simulink model "LKAS_AutoSave_DF_20211230_1703"  (R2018b)
settings: Solver=FixedStepDiscrete  StartTime=0.0  StopTime=10.0  FixedStep=0.01  RelTol=1e-3
InitFcn:
  | tmpVer = ver('MATLAB');
  | tmpVer = str2num(tmpVer.Version);
  | % -------------------------------------------------------------------
  | %  MATLAB file generated by Simulink.saveVars on 21-Nov-2019 10:06:14
  | %  MATLAB version: 7.13.0.564 (R2011b)
  | % -------------------------------------------------------------------
  | 
  | 
  | SInt16 = Simulink.AliasType;
  | SInt16.Description = 'Num';
  | if (tmpVer > 7.11)
  | 	SInt16.DataScope = 'Auto';
  | end
  | SInt16.HeaderFile = 'Rte_Type.h';
  | SInt16.BaseType = 'int16';
  | 
  | SInt32 = Simulink.AliasType;
  | SInt32.Description = 'Num';
  | if (tmpVer > 7.11)
  | 	SInt32.DataScope = 'Auto';
  | end
  | SInt32.HeaderFile = 'Rte_Type.h';
  | SInt32.BaseType = 'int32';
  | 
  | SInt8 = Simulink.AliasType;
  | SInt8.Description = 'Num';
  | if (tmpVer > 7.11)
  | 	SInt8.DataScope = 'Auto';
  | end
  | SInt8.HeaderFile = 'Rte_Type.h';
  | SInt8.BaseType = 'int8';
  | 
  | T_A_m2_1024_1_u32 = Simulink.NumericType;
  | T_A_m2_1024_1_u32.Description = 'm2 (square meters  (m2))';
  | if (tmpVer > 7.11)
  | 	T_A_m2_1024_1_u32.DataScope = 'Auto';
  | end
  | T_A_m2_1024_1_u32.HeaderFile = 'Rte_Type.h';
  | T_A_m2_1024_1_u32.DataTypeMode = 'Fixed-point: slope and bias scaling';
  | T_A_m2_1024_1_u32.SignednessBool = false;
  | T_A_m2_1024_1_u32.WordLength = 32;
  | T_A_m2_1024_1_u32.FixedExponent = -10;
  | T_A_m2_1024_1_u32.SlopeAdjustmentFactor = 1;
  | T_A_m2_1024_1_u32.Bias = 0;
  | T_A_m2_1024_1_u32.DataTypeOverride = 'Inherit';
  | T_A_m2_1024_1_u32.IsAlias = true;
  | 
  | T_A_m2_65536_1_u16 = Simulink.NumericType;
  | T_A_m2_65536_1_u16.Description = 'm2 (square meters  (m2))';
  | if (tmpVer > 7.11)
  | 	T_A_m2_65536_1_u16.DataScope = 'Auto';
  | end
  | T_A_m2_65536_1_u16.HeaderFile = 'Rte_Type.h';
  | T_A_m2_65536_1_u16.DataTypeMode = 'Fixed-point: slope and bias scaling';
  | T_A_m2_65536_1_u16.SignednessBool = false;
  | T_A_m2_65536_1_u16.WordLength = 16;
  | T_A_m2_65536_1_u16.FixedExponent = -16;
  | T_A_m2_65536_1_u16.SlopeAdjustmentFactor = 1;
  | T_A_m2_65536_1_u16.Bias = 0;
  | T_A_m2_65536_1_u16.DataTypeOverride = 'Inherit';
  | ... (+4647 lines)
StopFcn:
  | clear  T_A_m2_1024_1_u32 T_A_m2_65536_1_u16 T_A_m2_Float32 T_A_mm2_10_1_u16 T_A_mm2_4_1_s16 T_A_mm2_Float32 T_Cnt_Num_10_1_u32 T_Cnt_Num_1_1_s16 T_Cnt_Num_1_1_s32 T_Cnt_Num_1_1_s8 T_Cnt_Num_1_1_u16 T_Cnt_Num_1_1_u32 T_Cnt_Num_1_1_u8 T_E_J_1_1_s32 T_E_J_Float32 T_E_kJ_128_1_s32 T_E_kJ_Float32 T_E_kwh_10_1_u16 T_E_kwh_Float32 T_Epl_kwhpkm_100_1_u16 T_Epl_kwhpkm_Float32 T_F_N_1_1_s16 T_F_N_Float32 T_I_A_1000_1_u16 T_I_A_1048576_1_s32 T_I_A_2048_1_s16 T_I_A_32_1_s16 T_I_A_Float32 T_I_mA_1_1_s16 T_I_mA_32768_128_s16 T_I_mA_Float32 T_J_kgpm2_128_1_u16 T_J_kgpm2_Float32 T_K_NA_1000_1_s16 T_K_NA_100_1_s16 T_K_NA_100_1_u16 T_K_NA_1024_1_s16 T_K_NA_1024_1_u16 T_K_NA_128_1_s16 T_K_NA_128_1_u16 T_K_NA_128_1_u8 T_K_NA_16777216_1_u32 T_K_NA_16_1_s16 T_K_NA_16_1_u16 T_K_NA_16_1_u8 T_K_NA_1_16_u16 T_K_NA_1_1_s16 T_K_NA_1_1_u16 T_K_NA_1_1_u8 T_K_NA_32768_1_s16 T_K_NA_32768_1_u16 T_K_NA_32_1_s8 T_K_NA_4096_1_u16 T_K_NA_4194304_1_s32 T_K_NA_4194304_1_u16 T_K_NA_65536_1_s32 T_K_NA_65536_1_u16 T_K_NA_8192_1_s16 T_K_NA_8_1_s16 T_K_NA_Float32 T_M_Nm_16_1_s16 T_M_Nm_1_1_s16 T_M_Nm_32768_1_s16 T_M_Nm_32_1_s16 T_M_Nm_4_1_s16 T_M_Nm_512_1_s16 T_M_Nm_Float32 T_P_W_1_4_s16 T_P_W_1_8_s16 T_P_W_Float32 T_P_kW_128_1_s16 T_P_kW_1_8_s16 T_P_kW_8_1_s32 T_P_kW_Float32 T_Pct_pct_1024_1_s32 T_Pct_pct_1024_1_u32 T_Pct_pct_10_1_s16 T_Pct_pct_10_1_u32 T_Pct_pct_128_100_s8 T_Pct_pct_1_1_s16 T_Pct_pct_1_4_u8 T_Pct_pct_255_100_u16 T_Pct_pct_255_100_u8 T_Pct_pct_256_1_s16 T_Pct_pct_256_1_u16 T_Pct_pct_65535_100_u16 T_Pct_pct_Float32 T_R_ohm_1024_1_s16 T_R_ohm_32_1_s16 T_R_ohm_Float32 T_TK_K_16_1_s16 T_TK_K_Float32 T_T_degC_10_400_1_u16 T_T_degC_16_1_s16 T_T_degC_1_40_1_u8 T_T_degC_2_80_1_u8 T_T_degC_Float32 T_U_V_1000_1_u16 T_U_V_10_1_u8 T_U_V_200_1_u8 T_U_V_32_1_s16 T_U_V_4096_1_s16 T_U_V_512_1_s16 T_U_V_65535_8_u16 T_U_V_8192_1_u16 T_U_V_Float32 T_U_mV_1_1_s16 T_U_mV_256_20_u16 T_U_mV_Float32 T_V_l_256_1_s16 T_V_l_4096_1_s16 T_V_l_64_1_s16 T_V_l_65535_100_u16 T_V_l_Float32 T_V_ml_128_1_s16 T_V_ml_1_1_s16 T_V_ml_32768_1_s16 T_V_ml_Float32 T_V_ul_32_1_u16 T_V_ul_Float32 T_Vpl_clpkm_512_1_u16 T_Vpl_clpkm_Float32 T_a_kphps_16_1_s16 T_a_kphps_Float32 T_a_mps2_128_1_s16 T_a_mps2_Float32 T_c_MJpkg_256_1_s16 T_c_MJpkg_Float32 T_c_kJpgpK_1024_1_s16 T_c_kJpgpK_Float32 T_c_kJpkgpK_128_1_u16 T_c_kJpkgpK_Float32 T_chrg_Ah_1_1_s16 T_chrg_Ah_1_1_u16 T_chrg_Ah_1_1_u8 T_chrg_Ah_256_1_u16 T_chrg_Ah_4194304_1_s32 T_chrg_Ah_512_1_u16 T_chrg_Ah_8_1_u16 T_chrg_Ah_Float32 T_cmp_NA_100_1_s16 T_cmp_NA_128_1_s16 T_cmp_NA_16_1_s16 T_cmp_NA_32768_1_u16 T_cmp_NA_Float32 T_d2n_rpmps2_4_1_s16 T_d2n_rpmps2_Float32 T_dPct_pctps_16_1_s16 T_dPct_pctps_256_1_s16 T_dPct_pctps_Float32 T_dT_degCps_128_1_s16 T_dT_degCps_Float32 T_dV_lph_1_1_s16 T_dV_lph_Float32 T_dV_lpm_128_1_s16 T_dV_lpm_32_1_s16 T_dV_lpm_Float32 T_dV_lps_1024_1_u16 T_dV_lps_4_1_u16 T_dV_lps_Float32 T_dV_mlps_1024_1_s16 T_dV_mlps_Float32 T_d_BitField16 T_dm_gps_128_1_s16 T_dm_gps_128_1_u16 T_dm_gps_256_1_u16 T_dm_gps_Float32 T_dm_mgps_1_1_s16 T_dm_mgps_Float32 T_dn_rpmps_1_1_s16 T_dn_rpmps_2_1_s16 T_dn_rpmps_Float32 T_dp_Paps_1_1_s16 T_dp_Paps_Float32 T_dp_kPaps_1_1_s16 T_dp_kPaps_8_1_s16 T_dp_kPaps_Float32 T_dphi_degps_128_1_s16 T_dphi_degps_8_1_s16 T_dphi_degps_Float32 T_dr_ps_256_1_s16 T_dr_ps_Float32 T_drho_mgplps_1_2_s16 T_drho_mgplps_Float32 T_e_NA_1_1_u8 T_f_Hz_1_1_u16 T_f_Hz_1_1_u32 T_f_Hz_64_1_u16 T_f_Hz_8_1_s16 T_f_Hz_Float32 T_g_BitField32 T_l_km_16_1_s16 T_l_km_1_1_u16 T_l_km_1_1_u32 T_l_km_Float32 T_l_m_1024_1_s16 T_l_m_16_1_s16 T_l_m_1_1_u32 T_l_m_Float32 T_l_mm_16_1_s16 T_l_mm_1_1_u16 T_l_mm_4096_1_s16 T_l_mm_4_1_u8 T_l_mm_64_1_s16 T_l_mm_Float32 T_m_g_1_1_s16 T_m_g_2048_1_s16 T_m_g_32_1_u16 T_m_g_Float32 T_m_kg_1024_1_s16 T_m_kg_1_1_s16 T_m_kg_1_1_u32 T_m_kg_Float32 T_m_mg_128_1_s16 T_m_mg_32_1_s16 T_m_mg_Float32 T_n_rpm_1_1_s16 T_n_rpm_1_25_u8 T_n_rpm_256_50_u16 T_n_rpm_2_25_u8 T_n_rpm_4_1_u16 T_n_rpm_Float32 T_p_MPa_64_1_s16 T_p_MPa_Float32 T_p_Pa_1_1_s16 T_p_Pa_Float32 T_p_kPa_1_10_u16 T_p_kPa_1_1_s16 T_p_kPa_1_1_u8 T_p_kPa_256_1_u16 T_p_kPa_32_1_u16 T_p_kPa_64_1_s16 T_p_kPa_Float32 T_phi_deg_100_1_s16 T_phi_deg_1024_1_s16 T_phi_deg_128_1_s16 T_phi_deg_1_1_u8 T_phi_deg_256_1_s16 T_phi_deg_2_1_s8 T_phi_deg_32_1_s16 T_phi_deg_512_6_s32 T_phi_deg_Float32 T_phi_rad_2048_1_s16 T_phi_rad_Float32 T_r_NA_1024_1_s16 T_r_NA_1024_1_u16 T_r_NA_16384_1_s16 T_r_NA_16_1_s16 T_r_NA_256_1_s8 T_r_NA_256_1_u16 T_r_NA_32768_1_u16 T_r_NA_32_1_u16 T_r_NA_4096_1_s16 T_r_NA_65535_2_u16 T_r_NA_8192_1_u16 T_r_NA_Float32 T_rho_gpl_8192_1_s16 T_rho_gpl_Float32 T_rho_kgpm3_16_1_s16 T_rho_kgpm3_Float32 T_rho_mgpl_1_1_s16 T_rho_mgpl_64_1_s16 T_rho_mgpl_Float32 T_t_hour_1_1_s16 T_t_hour_Float32 T_t_m_1_1_u16 T_t_m_Float32 T_t_ms_1_1_s16 T_t_ms_1_1_u16 T_t_ms_1_1_u32 T_t_ms_4096_1_s16 T_t_ms_64_1_s16 T_t_ms_Float32 T_t_s_1000_1_s16 T_t_s_100_1_s16 T_t_s_10_1_s16 T_t_s_10_1_u16 T_t_s_1_1_s16 T_t_s_1_1_u16 T_t_s_1_1_u32 T_t_s_Float32 T_t_us_10_1_u32 T_t_us_1_1_s16 T_t_us_1_1_u32 T_t_us_1_4_u16 T_t_us_Float32 T_v_kph_1_1_u8 T_v_kph_64_1_s16 T_v_kph_64_1_u16 T_v_kph_Float32 T_v_mps_256_1_s16 T_v_mps_Float32 T_w_radps_32_1_s16 T_w_radps_Float32 T_y_BitField8 T_y_BitFieldDiagProgress T_y_BitFieldDiagStatus T_y_NA_1_1_u8 SInt16 SInt32 SInt8 T_BOOLEAN UInt16 UInt32 UInt8 s16 s32 s8 u16 u32 u8
model workspace (MAT data in the model file):
  MCOS : class17 (value not decoded)
  MCOS : class17 (value not decoded)
  MCOS : class17 (value not decoded)
  MCOS : class17 (value not decoded)
  MCOS : class17 (value not decoded)
  MCOS : class17 (value not decoded)
  MCOS : class17 (value not decoded)
  MCOS : class17 (value not decoded)
  MCOS : class17 (value not decoded)
  MCOS : class17 (value not decoded)
  MCOS : class17 (value not decoded)
  MCOS : class17 (value not decoded)
  MCOS : class17 (value not decoded)
  MCOS : class17 (value not decoded)
  MCOS : class17 (value not decoded)
  MCOS : class17 (value not decoded)
  MCOS : class17 (value not decoded)
  MCOS : class17 (value not decoded)
  MCOS : class17 (value not decoded)
  MCOS : class17 (value not decoded)
  MCOS : class17 (value not decoded)
  MCOS : class17 (value not decoded)
  MCOS : class17 (value not decoded)
  MCOS : class17 (value not decoded)
  MCOS : class17 (value not decoded)
  MCOS : class17 (value not decoded)
  MCOS : class17 (value not decoded)
  MCOS : class17 (value not decoded)
  MCOS : class17 (value not decoded)
  MCOS : class17 (value not decoded)
  MCOS : class17 (value not decoded)
  MCOS : class17 (value not decoded)
  MCOS : class17 (value not decoded)
  MCOS : class17 (value not decoded)
  MCOS : class17 (value not decoded)
  MCOS : class17 (value not decoded)
  MCOS : class17 (value not decoded)
  MCOS : class17 (value not decoded)
  MCOS : class17 (value not decoded)
  MCOS : class17 (value not decoded)
  MCOS : class17 (value not decoded)
  MCOS : class17 (value not decoded)
  MCOS : class17 (value not decoded)
  MCOS : class17 (value not decoded)
  MCOS : class17 (value not decoded)
  MCOS : class17 (value not decoded)
  MCOS : class17 (value not decoded)
  MCOS : class17 (value not decoded)
  MCOS : class17 (value not decoded)
  MCOS : class17 (value not decoded)
  MCOS : class17 (value not decoded)
  MCOS : class17 (value not decoded)
  MCOS : class17 (value not decoded)
  MCOS : class17 (value not decoded)
  MCOS : class17 (value not decoded)
  MCOS : class17 (value not decoded)
  MCOS : class17 (value not decoded)
  MCOS : class17 (value not decoded)
  MCOS : class17 (value not decoded)
  MCOS : class17 (value not decoded)
  MCOS : class17 (value not decoded)
  MCOS : class17 (value not decoded)
  MCOS : class17 (value not decoded)
  MCOS : class17 (value not decoded)
  MCOS : class17 (value not decoded)
  MCOS : class17 (value not decoded)
  MCOS : class17 (value not decoded)
  MCOS : class17 (value not decoded)
  MCOS : class17 (value not decoded)
  MCOS : class17 (value not decoded)
  MCOS : class17 (value not decoded)
  MCOS : class17 (value not decoded)
  MCOS : class17 (value not decoded)
  MCOS : class17 (value not decoded)
  MCOS : class17 (value not decoded)
  MCOS : class17 (value not decoded)
  MCOS : class17 (value not decoded)
  MCOS : class17 (value not decoded)
  MCOS : class17 (value not decoded)
  MCOS : class17 (value not decoded)
  MCOS : class17 (value not decoded)
  MCOS : class17 (value not decoded)
  MCOS : class17 (value not decoded)
  MCOS : class17 (value not decoded)
  MCOS : class17 (value not decoded)
  MCOS : class17 (value not decoded)
  MCOS : class17 (value not decoded)
  MCOS : class17 (value not decoded)
  MCOS : class17 (value not decoded)
  MCOS : class17 (value not decoded)
  MCOS : class17 (value not decoded)
  MCOS : class17 (value not decoded)
  MCOS : class17 (value not decoded)
  MCOS : class17 (value not decoded)
  MCOS : class17 (value not decoded)
  MCOS : class17 (value not decoded)
  MCOS : class17 (value not decoded)
undefined symbols (not defined in the file): LKA_CarWidth, LKA_SampleTime, LKA_StrRatio_C, LKA_Veh2CamL_C, LKA_Veh2CamW_C, LKA_WhlBaseL_C, LL_CompSWA_C, LL_CrvtPrvwT_C, LL_DesDvt_C, LL_DvtComp_C, LL_DvtPrvwT_C, LL_DvtSpdDet_vDvtSpdMin_C, LL_HdAgExT_C, LL_HdAgPrvwT_C, LL_LAccMax_C, LL_LAccRMax_C, LL_LDW_EarliestWarnLine_C, LL_LDW_LatestWarnLine_C, LL_LDWS_SUPPRESS_HEADING, LL_LFClb_TFC_FfCtlRatio_C, LL_LFClb_TFC_KdBalance_C, LL_LFClb_TFC_KdMaxSWA_C, LL_LFClb_TFC_KdV1_C, LL_LFClb_TFC_KdV2_C, LL_LFClb_TFC_KdVehSpdLwr_C, LL_LFClb_TFC_KdVehSpdUpr_C, LL_LFClb_TFC_Ki_C, LL_LFClb_TFC_KiMaxSWA_C, LL_LFClb_TFC_Kp_C, LL_LFClb_TFC_KpKlat_C, LL_LFClb_TFC_KpV1_C, LL_LFClb_TFC_KpV2_C, LL_LFClb_TFC_KpVehSpdLwr_C, LL_LFClb_TFC_KpVehSpdUpr_C, LL_LFClb_TFC_PrvwT_C, LL_LKA_EarliestWarnLine_C, LL_LKA_LatestWarnLine_C, LL_LKAExPrcs_ExitC0Dvt, LL_LKAExPrcs_ExitC0Swt, LL_LKAExPrcs_tiExitTime1, LL_LKAExPrcs_tiExitTime2, LL_LKAExPrcs_tiExitTime3, LL_LKAS_OUT_OF_CONTROL_LAT_VEL, LL_LKAS_OUT_OF_CONTROL_TTLC, LL_LKASWASyn_M0, LL_LKASWASyn_M1, LL_LKASWASyn_M2, LL_LKASWASyn_M3K, LL_LKASWASyn_SWAaddMax, LL_LKASWASyn_T2, LL_LKASWASyn_tiTrqSwaRtTime, LL_LKASWASyn_tiTrqSwaTime, LL_LKASWASyn_TrqMax, LL_LKASWASyn_TrqSwaAddSwt, LL_LKASWASyn_TrqSwaRateDiff, LL_LSpdCompT_C, LL_lStpLngth_C, LL_MAX_DELAY_EPSSTAR_TIME, LL_MAX_DRIVER_TORQUE_DISABLE, LL_MAX_DRIVER_TORQUE_ENABLE ... (+38)
libraries: simulink x138, canmsglib x8, dspstat3 x3, simulink_extras x1
(part 10 of 19)

== system LKAS_AutoSave_DF_20211230_1703/LKAS/LL/LLOn/LKA Input Processing (LKAInP)/Previewed Curvature Calculation (PrCrvt)/Curvature Ahead of Left Lane Line (CrvtAhdLft)1 ==
  CrvtAhdRgt_lPrvwDstZ : Inport
  CrvtAhdRgt_bsR0Info : Inport  Port=2
  Add : Sum  AccumDataTypeStr=single
  Bus Selector : BusSelector  OutputSignals=R0_C2,R0_C3
  Gain : Gain  Gain=2  OutDataTypeStr=single
  Gain1 : Gain  Gain=6  OutDataTypeStr=single
  Product : Product  OutDataTypeStr=single  RndMeth=Zero
  CrvtAhdRgt_crCrvtAhdRgt : Outport
  wires:
  Add/1 -> CrvtAhdRgt_crCrvtAhdRgt/1
  Product/1 -> Add/2
  Gain/1 -> Add/1
  Gain1/1 -> Product/1
  Bus Selector/1 -> Gain/1  "<R0_C2>"
  CrvtAhdRgt_lPrvwDstZ/1 -> Product/2
  Bus Selector/2 -> Gain1/1  "<R0_C3>"
  CrvtAhdRgt_bsR0Info/1 -> Bus Selector/1

== system LKAS_AutoSave_DF_20211230_1703/LKAS/LL/LLOn/LKA Input Processing (LKAInP)/Previewed Curvature Calculation (PrCrvt)/Lane Information Selection (LaneInfoSel) ==
  LaneInfoSel_stLKAActvFlg : Inport
  LaneInfoSel_facmLftLane : Inport  Port=2
  LaneInfoSel_facmRgtLane : Inport  Port=3
  If : If  IfExpression=u1==1  ElseIfExpressions=u1==2
  If Action Subsystem1 : Subsystem  TreatAsAtomicUnit=on
  If Action Subsystem2 : Subsystem  TreatAsAtomicUnit=on
  If Action Subsystem3 : Subsystem  TreatAsAtomicUnit=on
  Merge : Merge  Inputs=3
  LaneInfoSel_facmActvLane : Outport
  wires:
  If/3 -> If Action Subsystem3/Action
  If Action Subsystem3/1(Out1) -> Merge/3
  If Action Subsystem1/1(Out1) -> Merge/2
  If/2 -> If Action Subsystem1/Action
  Merge/1 -> LaneInfoSel_facmActvLane/1
  If Action Subsystem2/1(Out1) -> Merge/1
  If/1 -> If Action Subsystem2/Action
  LaneInfoSel_stLKAActvFlg/1 -> If/1
  LaneInfoSel_facmRgtLane/1 -> If Action Subsystem3/2(In2), If Action Subsystem1/1(In1)
  LaneInfoSel_facmLftLane/1 -> If Action Subsystem3/1(In1), If Action Subsystem2/1(In1)

== system LKAS_AutoSave_DF_20211230_1703/LKAS/LL/LLOn/LKA Input Processing (LKAInP)/Previewed Curvature Calculation (PrCrvt)/Z Calculation (ZCalc) ==
  ZCalc_vVehSpd : Inport
  ZCalc_tiCrvtPrvwT_C : Inport  Port=2
  Divide : Product  Inputs=**  OutDataTypeStr=single
  kph to mps : Gain  Gain=1/3.6  OutDataTypeStr=single
  ZCalc_lPrvwDstZ : Outport
  wires:
  Divide/1 -> ZCalc_lPrvwDstZ/1
  kph to mps/1 -> Divide/1
  ZCalc_tiCrvtPrvwT_C/1 -> Divide/2
  ZCalc_vVehSpd/1 -> kph to mps/1

== system LKAS_AutoSave_DF_20211230_1703/LKAS/LL/LLOn/LKA Input Processing (LKAInP)/Previewed Deviation Calculation (PrDvt)/Previewed Deviation of Left Lane Line (PrvwDvtLft) ==
  PrdcDvtLft_bsL0Info : Inport
  PrdcDvtLft_lPrvwDstZ : Inport  Port=2
  Add : Sum  Inputs=++++  AccumDataTypeStr=single
  Bus Selector : BusSelector  OutputSignals=L0_C0,L0_C1,L0_C2,L0_C3
  Product : Product  OutDataTypeStr=single  RndMeth=Zero
  Product3 : Product  OutDataTypeStr=single  RndMeth=Zero
  Product4 : Product  OutDataTypeStr=single  RndMeth=Zero
  Z*Z : Product  OutDataTypeStr=single  RndMeth=Zero
  Z*Z*Z : Product  OutDataTypeStr=single  RndMeth=Zero
  PrvwDvtLft_lPrvwDvtLft : Outport
  wires:
  Z*Z/1 -> Z*Z*Z/2, Product3/2
  Z*Z*Z/1 -> Product4/2
  Product4/1 -> Add/4
  Bus Selector/4 -> Product4/1  "<L0_C3>"
  Bus Selector/3 -> Product3/1  "<L0_C2>"
  Product3/1 -> Add/3
  Bus Selector/1 -> Add/1  "<L0_C0>"
  Product/1 -> Add/2
  Bus Selector/2 -> Product/1  "<L0_C1>"
  PrdcDvtLft_lPrvwDstZ/1 -> Z*Z/2, Product/2, Z*Z/1, Z*Z*Z/1
  PrdcDvtLft_bsL0Info/1 -> Bus Selector/1
  Add/1 -> PrvwDvtLft_lPrvwDvtLft/1

== system LKAS_AutoSave_DF_20211230_1703/LKAS/LL/LLOn/LKA Input Processing (LKAInP)/Previewed Deviation Calculation (PrDvt)/Previewed Deviation of Right Lane Line (PrvwDvtRgt) ==
  PrdcDvtRgt_lPrvwDstZ : Inport
  PrdcDvtRgt_bsR0Info : Inport  Port=2
  Add : Sum  Inputs=++++  AccumDataTypeStr=single
  Bus Selector : BusSelector  OutputSignals=R0_C0,R0_C1,R0_C2,R0_C3
  Product : Product  OutDataTypeStr=single  RndMeth=Zero
  Product3 : Product  OutDataTypeStr=single  RndMeth=Zero
  Product4 : Product  OutDataTypeStr=single  RndMeth=Zero
  Z*Z : Product  OutDataTypeStr=single  RndMeth=Zero
  Z*Z*Z : Product  OutDataTypeStr=single  RndMeth=Zero
  PrvwDvtRgt_lPrvwDvtRgt : Outport
  wires:
  Z*Z/1 -> Z*Z*Z/2, Product3/2
  Z*Z*Z/1 -> Product4/2
  Product4/1 -> Add/4
  Bus Selector/4 -> Product4/1  "<R0_C3>"
  Bus Selector/3 -> Product3/1  "<R0_C2>"
  Product3/1 -> Add/3
  Bus Selector/1 -> Add/1  "<R0_C0>"
  Add/1 -> PrvwDvtRgt_lPrvwDvtRgt/1
  Product/1 -> Add/2
  Bus Selector/2 -> Product/1  "<R0_C1>"
  PrdcDvtRgt_lPrvwDstZ/1 -> Z*Z/2, Product/2, Z*Z/1, Z*Z*Z/1
  PrdcDvtRgt_bsR0Info/1 -> Bus Selector/1

== system LKAS_AutoSave_DF_20211230_1703/LKAS/LL/LLOn/LKA Input Processing (LKAInP)/Previewed Deviation Calculation (PrDvt)/Z Calculation (ZCalc) ==
  ZCalc_vVehSpd : Inport
  ZCalc_tiDvtPrvwT_C : Inport  Port=2
  Divide : Product  Inputs=**  OutDataTypeStr=single
  kph to mps : Gain  Gain=1/3.6  OutDataTypeStr=single
  ZCalc_lPrvwDstZ : Outport
  wires:
  ZCalc_tiDvtPrvwT_C/1 -> Divide/2
  Divide/1 -> ZCalc_lPrvwDstZ/1
  kph to mps/1 -> Divide/1
  ZCalc_vVehSpd/1 -> kph to mps/1

== system LKAS_AutoSave_DF_20211230_1703/LKAS/LL/LLOn/LKA Input Processing (LKAInP)/Previewed Heading Angle Calculation (PrHdAg)/Perdicted Heading Angle from Right Lane Line (PrdcHdAgRgt) ==
  PrdcHdAgRgt_lPrvwDstZ : Inport
  PrdcHdAgRgt_bsR0Info : Inport  Port=2
  Add : Sum  Inputs=+++  AccumDataTypeStr=single
  Bus Selector : BusSelector  OutputSignals=R0_C1,R0_C2,R0_C3
  Gain : Gain  Gain=2  OutDataTypeStr=single
  Gain1 : Gain  Gain=3  OutDataTypeStr=single
  Product3 : Product  OutDataTypeStr=single  RndMeth=Zero
  Product4 : Product  OutDataTypeStr=single  RndMeth=Zero
  Z*Z : Product  OutDataTypeStr=single  RndMeth=Zero
  PrdcHdAgRgt_phiPrdcHdAgRgt : Outport
  wires:
  Gain1/1 -> Product4/1
  Gain/1 -> Product3/1
  Z*Z/1 -> Product4/2
  Product4/1 -> Add/3
  Bus Selector/3 -> Gain1/1  "<R0_C3>"
  Bus Selector/2 -> Gain/1  "<R0_C2>"
  Product3/1 -> Add/2
  Bus Selector/1 -> Add/1  "<R0_C1>"
  PrdcHdAgRgt_lPrvwDstZ/1 -> Z*Z/2, Product3/2, Z*Z/1
  PrdcHdAgRgt_bsR0Info/1 -> Bus Selector/1
  Add/1 -> PrdcHdAgRgt_phiPrdcHdAgRgt/1

== system LKAS_AutoSave_DF_20211230_1703/LKAS/LL/LLOn/LKA Input Processing (LKAInP)/Previewed Heading Angle Calculation (PrHdAg)/Perdicted Heading Angle from Right Lane Line (PrdcHdAgRgt)1 ==
  PrdcHdAgRgt_lPrvwDstZ : Inport
  PrdcHdAgRgt_bsR0Info : Inport  Port=2
  Add : Sum  Inputs=+++  AccumDataTypeStr=single
  Bus Selector : BusSelector  OutputSignals=R0_C1,R0_C2,R0_C3
  Gain : Gain  Gain=2  OutDataTypeStr=single
  Gain1 : Gain  Gain=3  OutDataTypeStr=single
  Product3 : Product  OutDataTypeStr=single  RndMeth=Zero
  Product4 : Product  OutDataTypeStr=single  RndMeth=Zero
  Z*Z : Product  OutDataTypeStr=single  RndMeth=Zero
  PrdcHdAgRgt_phiPrdcHdAgRgt : Outport
  wires:
  Gain1/1 -> Product4/1
  Gain/1 -> Product3/1
  Z*Z/1 -> Product4/2
  Product4/1 -> Add/3
  Bus Selector/3 -> Gain1/1  "<R0_C3>"
  Bus Selector/2 -> Gain/1  "<R0_C2>"
  Product3/1 -> Add/2
  Bus Selector/1 -> Add/1  "<R0_C1>"
  PrdcHdAgRgt_lPrvwDstZ/1 -> Z*Z/2, Product3/2, Z*Z/1
  PrdcHdAgRgt_bsR0Info/1 -> Bus Selector/1
  Add/1 -> PrdcHdAgRgt_phiPrdcHdAgRgt/1

== system LKAS_AutoSave_DF_20211230_1703/LKAS/LL/LLOn/LKA Input Processing (LKAInP)/Previewed Heading Angle Calculation (PrHdAg)/Predicted Heading Angle from Left Lane Line (PrdcHdAgtLft) ==
  PrdcHdAgtLft_bsL0Info : Inport
  PrdcHdAgtLft_lPrvwDstZ : Inport  Port=2
  Add : Sum  Inputs=+++  AccumDataTypeStr=single
  Bus Selector : BusSelector  OutputSignals=L0_C1,L0_C2,L0_C3
  Gain : Gain  Gain=2  OutDataTypeStr=single
  Gain1 : Gain  Gain=3  OutDataTypeStr=single
  Product3 : Product  OutDataTypeStr=single  RndMeth=Zero
  Product4 : Product  OutDataTypeStr=single  RndMeth=Zero
  Z*Z : Product  OutDataTypeStr=single  RndMeth=Zero
  PrdcHdAgtLft_phiPrdcHdAgLft : Outport
  wires:
  Gain1/1 -> Product4/1
  Gain/1 -> Product3/1
  Z*Z/1 -> Product4/2
  Product4/1 -> Add/3
  Bus Selector/3 -> Gain1/1  "<L0_C3>"
  Bus Selector/2 -> Gain/1  "<L0_C2>"
  Product3/1 -> Add/2
  Bus Selector/1 -> Add/1  "<L0_C1>"
  PrdcHdAgtLft_lPrvwDstZ/1 -> Z*Z/2, Product3/2, Z*Z/1
  PrdcHdAgtLft_bsL0Info/1 -> Bus Selector/1
  Add/1 -> PrdcHdAgtLft_phiPrdcHdAgLft/1

== system LKAS_AutoSave_DF_20211230_1703/LKAS/LL/LLOn/LKA Input Processing (LKAInP)/Previewed Heading Angle Calculation (PrHdAg)/Predicted Heading Angle from Left Lane Line (PrdcHdAgtLft)1 ==
  PrdcHdAgtLft_bsL0Info : Inport
  PrdcHdAgtLft_lPrvwDstZ : Inport  Port=2
  Add : Sum  Inputs=+++  AccumDataTypeStr=single
  Bus Selector : BusSelector  OutputSignals=L0_C1,L0_C2,L0_C3
  Gain : Gain  Gain=2  OutDataTypeStr=single
  Gain1 : Gain  Gain=3  OutDataTypeStr=single
  Product3 : Product  OutDataTypeStr=single  RndMeth=Zero
  Product4 : Product  OutDataTypeStr=single  RndMeth=Zero
  Z*Z : Product  OutDataTypeStr=single  RndMeth=Zero
  PrdcHdAgtLft_phiPrdcHdAgLft : Outport
  wires:
  Gain1/1 -> Product4/1
  Gain/1 -> Product3/1
  Z*Z/1 -> Product4/2
  Product4/1 -> Add/3
  Bus Selector/3 -> Gain1/1  "<L0_C3>"
  Bus Selector/2 -> Gain/1  "<L0_C2>"
  Product3/1 -> Add/2
  Bus Selector/1 -> Add/1  "<L0_C1>"
  PrdcHdAgtLft_lPrvwDstZ/1 -> Z*Z/2, Product3/2, Z*Z/1
  PrdcHdAgtLft_bsL0Info/1 -> Bus Selector/1
  Add/1 -> PrdcHdAgtLft_phiPrdcHdAgLft/1

== system LKAS_AutoSave_DF_20211230_1703/LKAS/LL/LLOn/LKA Input Processing (LKAInP)/Previewed Heading Angle Calculation (PrHdAg)/Z Calculation (ZCalc) ==
  ZCalc_vVehSpd : Inport
  ZCalc_tiHdAgPrvwT_C : Inport  Port=2
  Divide : Product  Inputs=**  OutDataTypeStr=single
  kph to mps : Gain  Gain=1/3.6  OutDataTypeStr=single
  ZCalc_lPrvwDstZ : Outport
  wires:
  kph to mps/1 -> Divide/1
  Divide/1 -> ZCalc_lPrvwDstZ/1
  ZCalc_tiHdAgPrvwT_C/1 -> Divide/2
  ZCalc_vVehSpd/1 -> kph to mps/1

== system LKAS_AutoSave_DF_20211230_1703/LKAS/LL/LLOn/LKA Input Processing (LKAInP)/Previewed Heading Angle Calculation (PrHdAg)/Z Calculation (ZCalc)1 ==
  ZCalc_vVehSpd : Inport
  ZCalc_tiHdAgPrvwT_C : Inport  Port=2
  Divide : Product  Inputs=**  OutDataTypeStr=single
  kph to mps : Gain  Gain=1/3.6  OutDataTypeStr=single
  ZCalc_lPrvwDstZ : Outport
  wires:
  kph to mps/1 -> Divide/1
  Divide/1 -> ZCalc_lPrvwDstZ/1
  ZCalc_tiHdAgPrvwT_C/1 -> Divide/2
  ZCalc_vVehSpd/1 -> kph to mps/1

== system LKAS_AutoSave_DF_20211230_1703/LKAS/LL/LLOn/LKA Input Processing (LKAInP)/Steering Wheel Position Calculation (SWAPosCal)/Subsystem ==
  SWAIn : Inport
  LKA_SampleTime : Inport  Port=2
  Enable : EnablePort
      settings: AttributesFormatString=states = %<StatesWhenEnabling>
  Constant : Constant  Value=10  OutDataTypeStr=single
  LowPass : Subsystem
  Saturation : Saturate  UpperLimit=3  LowerLimit=-3
      settings: AttributesFormatString="Min = %<LowerLimit>  Max = %<UpperLimit>"
  SWAPos : Outport  InitialOutput=0
      settings: AttributesFormatString=%<OutputWhenDisabled> = %<InitialOutput>
  wires:
  SWAIn/1 -> LowPass/2(u)
  LowPass/1(y) -> Saturation/1  "SWAPos"
  Constant/1 -> LowPass/1(T)
  LKA_SampleTime/1 -> LowPass/3(dT)
  Saturation/1 -> SWAPos/1

== system LKAS_AutoSave_DF_20211230_1703/LKAS/LL/LLOn/LKA Input Processing (LKAInP)/Steering Wheel Position Calculation (SWAPosCal)/Subsystem1 ==
  L0 : Inport
  R0 : Inport  Port=2
  VehSpd : Inport  Port=3
  SWA : Inport  Port=4
  LKA_SampleTime : Inport  Port=5
  Abs{2,4..7} (5 alike) : Abs
  Bus Selector : BusSelector  OutputSignals=L0_C1,L0_C2,L0_Q
  Bus Selector1 : BusSelector  OutputSignals=R0_C1,R0_C2,R0_Q
  Compare To Constant : simulink/Logic and Bit Operations/Compare To Constant  relop===  const=3.0  OutDataTypeStr=boolean
  Compare To Constant1 : simulink/Logic and Bit Operations/Compare To Constant  relop===  const=3.0  OutDataTypeStr=boolean
  Constant : Constant  Value=0.0001  OutDataTypeStr=single
  Constant1 : Constant  Value=0.005  OutDataTypeStr=single
  Constant3 : Constant  Value=2  OutDataTypeStr=single
  Constant4 : Constant  Value=50  OutDataTypeStr=single
  Constant5 : Constant  OutDataTypeStr=single
  Divide : Product  Inputs=*/
  Logical Operator : Logic  AllPortsSameDT=off  OutDataTypeStr=boolean
  Logical Operator1 : Logic  AllPortsSameDT=off  OutDataTypeStr=boolean
  Logical Operator3 : Logic  Inputs=5  AllPortsSameDT=off  OutDataTypeStr=boolean
  Logical Operator4 : Logic  AllPortsSameDT=off  OutDataTypeStr=boolean
  Relational Operator{,1..3,7} (5 alike) : RelationalOperator  Operator=<=  OutDataTypeStr=boolean  RndMeth=Simplest
  Relational Operator6 : RelationalOperator  OutDataTypeStr=boolean  RndMeth=Simplest
  Subsystem : Subsystem
  Flg : Outport
  wires:
  L0/1 -> Bus Selector/1
  R0/1 -> Bus Selector1/1
  Logical Operator1/1 -> Logical Operator3/1
  Bus Selector/3 -> Compare To Constant/1  "<L0_Q>"
  Abs2/1 -> Relational Operator7/1
  Bus Selector1/3 -> Compare To Constant1/1  "<R0_Q>"
  Relational Operator2/1 -> Logical Operator1/1
  Compare To Constant1/1 -> Logical Operator4/2
  Relational Operator6/1 -> Logical Operator3/4
  Abs7/1 -> Relational Operator3/1
  Constant1/1 -> Relational Operator3/2, Relational Operator2/2
  Constant/1 -> Relational Operator1/2, Relational Operator/2
  Abs4/1 -> Relational Operator/1
  Constant3/1 -> Divide/1
  Logical Operator3/1 -> Subsystem/Enable, Subsystem/1(In)  "SWA"
  VehSpd/1 -> Relational Operator6/1
  Constant4/1 -> Relational Operator6/2
  Abs6/1 -> Relational Operator2/1
  Compare To Constant/1 -> Logical Operator4/1
  Relational Operator7/1 -> Logical Operator3/5
  Bus Selector1/2 -> Abs5/1  "<R0_C2>"
  Abs5/1 -> Relational Operator1/1
  Relational Operator1/1 -> Logical Operator/2
  Relational Operator3/1 -> Logical Operator1/2
  SWA/1 -> Abs2/1
  Logical Operator/1 -> Logical Operator3/2
  Constant5/1 -> Relational Operator7/2
  Subsystem/1(Out) -> Flg/1
  Bus Selector/1 -> Abs6/1  "<L0_C1>"
  Bus Selector1/1 -> Abs7/1  "<R0_C1>"
  Logical Operator4/1 -> Logical Operator3/3
  Bus Selector/2 -> Abs4/1  "<L0_C2>"
  Divide/1 -> Subsystem/2(In1)
  Relational Operator/1 -> Logical Operator/1
  LKA_SampleTime/1 -> Divide/2

== system LKAS_AutoSave_DF_20211230_1703/LKAS/LL/LLOn/LKA Input Processing (LKAInP)/Under The Limit (UndrLim)/Steering Wheel Angel Max (SWAMax) ==
  SWAMax_vVehSpd : Inport
  SWAMax_aLAcc_C : Inport  Port=2
  LKA_StrRatio_C : Inport  Port=3
  LKA_WhlBaseL_C : Inport  Port=4
  Constant : Constant  Value=0.09  OutDataTypeStr=single
  Divide1 : Product  Inputs=*/
  MATLAB Function : MATLAB Function  TreatAsAtomicUnit=on
  Saturation1 : Saturate  UpperLimit=0.0117  LowerLimit=0.00237
      settings: AttributesFormatString="Min = %<LowerLimit>  Max = %<UpperLimit>"
  Saturation3 : Saturate  UpperLimit=150  LowerLimit=60
      settings: AttributesFormatString="Min = %<LowerLimit>  Max = %<UpperLimit>"
  kph To mps : Gain  Gain=1/3.6  OutDataTypeStr=single
  SWAMax_phiSWAMax : Outport
  wires:
  LKA_StrRatio_C/1 -> MATLAB Function/3(i)
  LKA_WhlBaseL_C/1 -> MATLAB Function/4(L)
  kph To mps/1 -> MATLAB Function/1(v)
  SWAMax_vVehSpd/1 -> Saturation3/1, kph To mps/1
  Divide1/1 -> Saturation1/1
  Saturation1/1 -> MATLAB Function/5(K)
  SWAMax_aLAcc_C/1 -> MATLAB Function/2(ax)
  MATLAB Function/1(SWAmax) -> SWAMax_phiSWAMax/1
  Constant/1 -> Divide1/1
  Saturation3/1 -> Divide1/2  "Vx"

== system LKAS_AutoSave_DF_20211230_1703/LKAS/LL/LLOn/LKA Input Processing (LKAInP)/Under The Limit (UndrLim)/Steering Wheel Angel Rate Max (SWARMax) ==
  SWARateMax_vVehSpd : Inport
  SWARateMax_aLAccR_C : Inport  Port=2
  LKA_StrRatio_C : Inport  Port=3
  LKA_WhlBaseL_C : Inport  Port=4
  Constant : Constant  Value=0.09  OutDataTypeStr=single
  Divide1 : Product  Inputs=*/
  MATLAB Function : MATLAB Function  TreatAsAtomicUnit=on
  Saturation1 : Saturate  UpperLimit=0.0117  LowerLimit=0.00237
      settings: AttributesFormatString="Min = %<LowerLimit>  Max = %<UpperLimit>"
  Saturation3 : Saturate  UpperLimit=150  LowerLimit=60
      settings: AttributesFormatString="Min = %<LowerLimit>  Max = %<UpperLimit>"
  kph To mps : Gain  Gain=1/3.6  OutDataTypeStr=single
  SWARMax_dphiSWARMax : Outport
  wires:
  kph To mps/1 -> MATLAB Function/1(v)
  LKA_WhlBaseL_C/1 -> MATLAB Function/4(L)
  LKA_StrRatio_C/1 -> MATLAB Function/3(i)
  MATLAB Function/1(SWARmax) -> SWARMax_dphiSWARMax/1
  SWARateMax_vVehSpd/1 -> Saturation3/1, kph To mps/1
  Divide1/1 -> Saturation1/1
  Saturation1/1 -> MATLAB Function/5(K)
  SWARateMax_aLAccR_C/1 -> MATLAB Function/2(dax)
  Constant/1 -> Divide1/1
  Saturation3/1 -> Divide1/2  "Vx"

== system LKAS_AutoSave_DF_20211230_1703/LKAS/LL/LLOn/LL State Determination (LLStateDet)/LL State Machine Conditions (LLSMCon)/Activation Condition (ActvC) ==
  DACMode : Inport
  InInfoSyn : Inport  Port=2
  LKAInPInfo : Inport  Port=3
  LLClb : Inport  Port=4
  Activation Condition Synthesis (ActvCSyn) : Subsystem  Description=|
      | Block Name: Activation Condition Synthesis
      | Ab.: ActvCSyn
      | No.: 1.1.1.4.4
      | Rev: 0.0.1
      | Update Date: 19-3-26
  Bus Selector : BusSelector  OutputSignals=bsEPSInfo,bsLaneInfo.bsL0Info.L0_Q,bsLaneInfo.bsR0Info.R0_Q
  Bus Selector1 : BusSelector  OutputSignals=LaneWidth,bsDvtInfo.ILftDvt,bsDvtInfo.IRgtDvt
  Deviation Threshold Condition (DvtThresCon) : Subsystem
  EPS Controllability Enable Condition (EPSCtlEC) : Subsystem  Description=|
      | Block Name: EPS Controllability Enable Condition
      | Ab.: EPSCtlEC
      | No.: 1.1.1.4.1
      | Rev: 0.0.1
      | Update Date: 19-3-26
  Lane Quality Enable Condition (LaneQlEC) : Subsystem  Description=|
      | Block Name: Lane Quality Enable Condition
      | Ab.: LaneQlEC
      | No.: 1.1.1.4.3
      | Rev: 0.0.1
      | Update Date: 19-3-26
  ActvC_stLDWActvCSyn : Outport
  ActvC_stLKAActvCSyn : Outport  Port=2
  wires:
  InInfoSyn/1 -> Bus Selector/1, Deviation Threshold Condition (DvtThresCon)/5(DvtThresCon_InInfoSyn)
  Activation Condition Synthesis (ActvCSyn)/1(ActvCSyn_stLDWActvCSyn) -> ActvC_stLDWActvCSyn/1
  Deviation Threshold Condition (DvtThresCon)/2(DvtThresCon_stDvtThresActvFlgLKA) -> Activation Condition Synthesis (ActvCSyn)/4(ActvCSyn_stDvtThresActvFlgLKA), Lane Quality Enable Condition (LaneQlEC)/1(LaneQlEC_stDvtThresActvFlg)
  Bus Selector/1 -> EPS Controllability Enable Condition (EPSCtlEC)/1(EPSCtlEC_bsEPSInfo)  "<bsEPSInfo>"
  Bus Selector/2 -> Lane Quality Enable Condition (LaneQlEC)/2(LaneQlEC_stFacmL0Ql)  "<L0_Q>"
  Bus Selector/3 -> Lane Quality Enable Condition (LaneQlEC)/3(LaneQlEC_stFacmR0Ql)  "<R0_Q>"
  DACMode/1 -> Activation Condition Synthesis (ActvCSyn)/1(ActvCSyn_stDACMode)
  EPS Controllability Enable Condition (EPSCtlEC)/1(EPSCtlEC_stEPSCtlEC) -> Activation Condition Synthesis (ActvCSyn)/2(ActvCSyn_stEPSCtlEC)  "ACTIVE_EPS"
  Lane Quality Enable Condition (LaneQlEC)/1(LaneQlEC_stLaneQlECFlgLKA) -> Activation Condition Synthesis (ActvCSyn)/5(ActvCSyn_stLaneQlECFlg)  "ACTIVE_LANEQUALITY"
  Activation Condition Synthesis (ActvCSyn)/2(ActvCSyn_stLKAActvCSyn) -> ActvC_stLKAActvCSyn/1  "ACTIVE"
  LLClb/1 -> Deviation Threshold Condition (DvtThresCon)/4(DvtThresCon_bsDvtThresClb)
  Deviation Threshold Condition (DvtThresCon)/1(DvtThresCon_stDvtThresActvFlgLDW) -> Activation Condition Synthesis (ActvCSyn)/3(ActvCSyn_stDvtThresActvFlgLDW)
  LKAInPInfo/1 -> Bus Selector1/1
  Bus Selector1/2 -> Deviation Threshold Condition (DvtThresCon)/2(DvtThresCon_ILftDvt)  "<ILftDvt>"
  Bus Selector1/3 -> Deviation Threshold Condition (DvtThresCon)/3(DvtThresCon_IRgtDvt)  "<IRgtDvt>"
  Bus Selector1/1 -> Deviation Threshold Condition (DvtThresCon)/1(DvtThresCon_lLaneWidth)  "<LaneWidth>"

== system LKAS_AutoSave_DF_20211230_1703/LKAS/LL/LLOn/LL State Determination (LLStateDet)/LL State Machine Conditions (LLSMCon)/Deactivation Condition (DeactvC) ==
  DACMode : Inport
  InInfoSyn : Inport  Port=2
  LKAInPInfo : Inport  Port=3
  LLClb : Inport  Port=4
  LLState : Inport  Port=5
  ExitFlg : Inport  Port=6
  Bus Selector : BusSelector  OutputSignals=bsVehMovInfo.ESC_VehSpd,bsEPSInfo
  Bus Selector1 : BusSelector  OutputSignals=LaneWidth,bsDvtInfo.ILftDvt,bsDvtInfo.IRgtDvt,bsPrCrvtInfo.crPrvwCrvt
  Deactivation Condition Synthesis (DeactvCSyn) : Subsystem  Description=|
      | Block Name: Deactivation Condition Synthesis
      | Ab.: DeactvCSyn
      | No.: 1.1.1.5.3
      | Rev: 0.0.1
      | Update Date: 19-3-26
  Deviation Threshold Condition (DvtThresCon) : Subsystem
  Driver Take Condition (DvrTkCon) : Subsystem  Description=|
      | Block Name: EPS Condition
      | Ab.: EPSC
      | No.: 1.1.1.5.2
      | Rev: 0.0.1
      | Update Date: 19-3-26
  EPS Condition (EPSC) : Subsystem  Description=|
      | Block Name: EPS Condition
      | Ab.: EPSC
      | No.: 1.1.1.5.2
      | Rev: 0.0.1
      | Update Date: 19-3-26
  DeactvC_stLDWDeactvCSyn : Outport
  DeactvC_stLKADeactvCSyn : Outport  Port=2
  wires:
  InInfoSyn/1 -> Bus Selector/1, Deviation Threshold Condition (DvtThresCon)/5(DvtThresCon_InInfoSyn)
  Deactivation Condition Synthesis (DeactvCSyn)/1(DeactvCSyn_stLDWDeactvCSyn) -> DeactvC_stLDWDeactvCSyn/1
  LLClb/1 -> EPS Condition (EPSC)/1(EPSC_bsLLClb), Driver Take Condition (DvrTkCon)/3(DvrTkCon_bsLLClb), Deviation Threshold Condition (DvtThresCon)/4(DvtThresCon_bsDvtThresClb)
  Deviation Threshold Condition (DvtThresCon)/2(DvtThresCon_stDvtThresActvFlgLKA) -> Driver Take Condition (DvrTkCon)/2(DvrTkCon_stActvFlg), Deactivation Condition Synthesis (DeactvCSyn)/3(DeactvCSyn_stDvtThresActvFlgLKA)
  LLState/1 -> EPS Condition (EPSC)/3(EPSC_bsLLState)
  Bus Selector/2 -> Driver Take Condition (DvrTkCon)/5(DvrTkCon_bsEPSInfo), EPS Condition (EPSC)/2(EPSC_bsEPSInfo)  "<bsEPSInfo>"
  EPS Condition (EPSC)/1(EPSC_stEPSCFlg) -> Deactivation Condition Synthesis (DeactvCSyn)/5(DeactvCSyn_stEPSCFlg)
  ExitFlg/1 -> Deactivation Condition Synthesis (DeactvCSyn)/6(DeactvCSyn_stExitFlg)
  DACMode/1 -> Deactivation Condition Synthesis (DeactvCSyn)/1(DeactvCSyn_stDACMode)
  Deactivation Condition Synthesis (DeactvCSyn)/2(DeactvCSyn_stLKADeactvCSyn) -> DeactvC_stLKADeactvCSyn/1  "DEACTIVE"
  Bus Selector/1 -> Driver Take Condition (DvrTkCon)/4(DvrTkCon_vVehSpd)  "<ESC_VehSpd>"
  Driver Take Condition (DvrTkCon)/1(DvrTkCon_stDvrTkConFlg) -> Deactivation Condition Synthesis (DeactvCSyn)/4(DvrTkCon_stDvrTkConFlg)
  LKAInPInfo/1 -> Bus Selector1/1
  Bus Selector1/3 -> Deviation Threshold Condition (DvtThresCon)/3(DvtThresCon_IRgtDvt)  "<IRgtDvt>"
  Bus Selector1/2 -> Deviation Threshold Condition (DvtThresCon)/2(DvtThresCon_ILftDvt)  "<ILftDvt>"
  Bus Selector1/4 -> Driver Take Condition (DvrTkCon)/1(DvrTkCon_crPrvwCrvt)  "<crPrvwCrvt>"
  Bus Selector1/1 -> Deviation Threshold Condition (DvtThresCon)/1(DvtThresCon_lLaneWidth)  "<LaneWidth>"
  Deviation Threshold Condition (DvtThresCon)/1(DvtThresCon_stDvtThresActvFlgLDW) -> Deactivation Condition Synthesis (DeactvCSyn)/2(DeactvCSyn_stDvtThresActvFlgLDW)

== system LKAS_AutoSave_DF_20211230_1703/LKAS/LL/LLOn/LL State Determination (LLStateDet)/LL State Machine Conditions (LLSMCon)/Disable Condition (DisblC) ==
  DACMode : Inport
  InInfoSyn : Inport  Port=2
  LKAInPInfo : Inport  Port=3
  LLClb : Inport  Port=4
  LLState : Inport  Port=5
  Bus Selector : BusSelector  OutputSignals=LaneWidth,bsPrCrvtInfo.crPrvwCrvt,bsTTLCInfo,bsDvtInfo
  Disable Condition Synthesis (DisblCSyn) : Subsystem  Description=|
      | Block Name: Disable Condition Synthesis
      | Ab.: DisblCSyn
      | No.: 1.1.1.3.8.0
      | Rev: 0.0.1
      | Update Date: 19-3-26
  Driver Intent Condition (DrvInttC) : Subsystem  Description=|
      | Block Name: Driver Intent Condition
      | Ab.: DrvInttC
      | No.: 1.1.1.3.3.0
      | Rev: 0.0.1
      | Update Date: 19-3-26
  LDW Alarm Timeout (LDWAlrmTOut) : Subsystem  Description=|
      | Block Name: LDW Alarm Timeout
      | Ab.: LDWAlrmTOut
      | No.: 1.1.1.3.6.0
      | Rev: 0.0.1
      | Update Date: 19-3-26
  LDW Own Condition (LDWOwnC) : Subsystem  Description=|
      | Block Name: LDW Own Condition
      | Ab.: LDWOwnC
      | No.: 1.1.1.3.4.0
      | Rev: 0.0.1
      | Update Date: 19-3-26
  LKA Own Condition (LKAOwnC) : Subsystem  Description=|
      | Block Name: LKA Own Condition
      | Ab.: LKAOwnC
      | No.: 1.1.1.3.5.0
      | Rev: 0.0.1
      | Update Date: 19-3-26
  Lane Condition (LaneC) : Subsystem  Description=|
      | Block Name: Lane Condition
      | Ab.: LaneC
      | No.: 1.1.1.3.2.0
      | Rev: 0.0.1
      | Update Date: 19-3-26
  Subsystem : Subsystem  Commented=on
  Subsystem1 : Subsystem
  Vehicle State Condition (VehStateC) : Subsystem  Description=|
      | Block Name: Vehicle State Condition
      | Ab.: VehStateC
      | No.: 1.1.1.3.1.0
      | Rev: 0.0.1
      | Update Date: 19-3-26
  DisblC_stLDWDisblCSyn : Outport
  DisblC_stLKADisblCSyn : Outport  Port=2
  Disable_Reason : Outport  Port=3
  wires:
  Vehicle State Condition (VehStateC)/1(VehStateC_stVehStateCSyn) -> Disable Condition Synthesis (DisblCSyn)/2(DisblCSyn_stVehStateC)
  Lane Condition (LaneC)/1(LaneC_stLanCSyn) -> Disable Condition Synthesis (DisblCSyn)/3(DisblCSyn_stLaneC)
  Driver Intent Condition (DrvInttC)/1(DrvInttC_stDrvInttCSyn) -> Disable Condition Synthesis (DisblCSyn)/4(DisblCSyn_stDrvInttC)
  LDW Own Condition (LDWOwnC)/1(LDWOwnC_stLDWOwnCSyn) -> Subsystem1/4(LDWOwnCSyn), Disable Condition Synthesis (DisblCSyn)/5(DisblCSyn_stLDWOwnC)  "LDWOwnCSyn"
  LKA Own Condition (LKAOwnC)/1(LKAOwnC_stLKAOwnCSyn) -> Disable Condition Synthesis (DisblCSyn)/6(DisblCSyn_stLKAOwnC)
  Disable Condition Synthesis (DisblCSyn)/1(DisblCSyn_stLDWDisblCSyn) -> DisblC_stLDWDisblCSyn/1
  LLState/1 -> LDW Alarm Timeout (LDWAlrmTOut)/1(LDWAlrmTOut_bsLLState), LKA Own Condition (LKAOwnC)/4(LKAOwnC_bsLLState)
  LLClb/1 -> Vehicle State Condition (VehStateC)/3(VehStateC_bsLLClb), LDW Alarm Timeout (LDWAlrmTOut)/2(LDWAlrmTOut_bsLLClb), LKA Own Condition (LKAOwnC)/5(LKAOwnC_bsLLClb), LDW Own Condition (LDWOwnC)/3(LDWOwnC_bsLLClb), Driver Intent Condition (DrvInttC)/2(DrvInttC_bsLLClb), Lane Condition (LaneC)/4(LaneC_bsLLClb)
  DACMode/1 -> Vehicle State Condition (VehStateC)/1(VehStateC_stDACMode), LKA Own Condition (LKAOwnC)/1(LKAOwnC_stDACMode), LDW Own Condition (LDWOwnC)/1(LDWOwnC_stDACMode), Disable Condition Synthesis (DisblCSyn)/1(DisblCSyn_stDACMode)
  LDW Alarm Timeout (LDWAlrmTOut)/1(LDWAlrmTOut_stLDWAlrmTOut) -> Subsystem1/6(LDWAlrmTOut), Disable Condition Synthesis (DisblCSyn)/7(DisblCSyn_stLDWAlrmTOut)  "LDWAlrmTOut"
  InInfoSyn/1 -> Vehicle State Condition (VehStateC)/2(VehStateC_bsInInfoSyn), LKA Own Condition (LKAOwnC)/2(LKAOwnC_bsInInfoSyn), Driver Intent Condition (DrvInttC)/1(DrvInttC_bsInInfoSyn), Lane Condition (LaneC)/1(LaneC_bsInInfoSyn)
  Disable Condition Synthesis (DisblCSyn)/2(DisblCSyn_stLKADisblCSyn) -> DisblC_stLKADisblCSyn/1  "DISABLE"
  LKA Own Condition (LKAOwnC)/2(LKAOwnC) -> Subsystem1/5(LKAOwnCSyn)  "LKAOwnSyn"
  Driver Intent Condition (DrvInttC)/2(DrvInttCSyn) -> Subsystem1/3(DrvInttCSyn)  "DrvInttCSyn"
  Lane Condition (LaneC)/2(LanCSyn) -> Subsystem1/2(LanCSyn)  "LaneCSyn"
  Vehicle State Condition (VehStateC)/2(VehStateC) -> Subsystem1/1(VehStateC)  "VehStateC"
  LKAInPInfo/1 -> Bus Selector/1
  Bus Selector/3 -> LKA Own Condition (LKAOwnC)/3(LKAOwnC_bsTTLCInfo)  "<bsTTLCInfo>"
  Bus Selector/2 -> Driver Intent Condition (DrvInttC)/3(DrvInttC_crPrvwCrvt), Lane Condition (LaneC)/3(LaneC_crPrvwCrvt)  "<crPrvwCrvt>"
  Bus Selector/1 -> Lane Condition (LaneC)/2(LaneC_LaneWidth)  "<LaneWidth>"
  Bus Selector/4 -> LKA Own Condition (LKAOwnC)/6(LKAOwnC_bsDvtInfo), LDW Own Condition (LDWOwnC)/2(LDWOwnC_bsPrDvtInfo)  "<bsDvtInfo>"
  Subsystem1/1(DisableReason) -> Disable_Reason/1

== system LKAS_AutoSave_DF_20211230_1703/LKAS/LL/LLOn/LL State Determination (LLStateDet)/LL State Machine Conditions (LLSMCon)/Enable Condition (EnaC) ==
  EnaC_stDACMode : Inport
  EnaC_bsInInfoSyn : Inport  Port=2
  EnaC_bsLKAInPInfo : Inport  Port=3
  EnaC_bsLLClb : Inport  Port=4
  Bus Selector : BusSelector  OutputSignals=LaneWidth,bsPrCrvtInfo.crPrvwCrvt,bsTTLCInfo,bsDvtInfo
  Driver Intent Condition (DrvInttC) : Subsystem  Description=|
      | Block Name: Driver Intent Condition
      | Ab.: DrvInttC
      | No.: 1.1.1.2.3.0
      | Rev: 0.0.1
      | Update Date: 19-3-26
  Enable Condition Synthesis (EnaCSyn) : Subsystem  Description=|
      | Block Name: Enable Condition Synthesis
      | Ab.: EnaCSyn
      | No.: 1.1.1.2.7.0
      | Rev: 0.0.1
      | Update Date: 19-3-26
  LDW Own Condition (LDWOwnC) : Subsystem  Description=|
      | Block Name: LDW Own Condition
      | Ab.: LDWOwnC
      | No.: 1.1.1.2.4.0
      | Rev: 0.0.1
      | Update Date: 19-3-26
  LKA Own Condition (LKAOwnC) : Subsystem  Description=|
      | Block Name: LKA Own Condition
      | Ab.: LKAOwnC
      | No.: 1.1.1.2.5.0
      | Rev: 0.0.1
      | Update Date: 19-3-26
  Lane Condition (LaneC) : Subsystem  Description=|
      | Block Name: Lane Condition
      | Ab.: LaneC
      | No.: 1.1.1.2.2.0
      | Rev: 0.0.1
      | Update Date: 19-3-26
  Vehicle State Condition (VehStateC) : Subsystem  Description=|
      | Block Name: Vehicle State Condition
      | Ab.: VehStateC
      | No.: 1.1.1.2.1.0
      | Rev: 0.0.1
      | Update Date: 19-3-26
  EnaC_stLDWEnaCSyn : Outport
  EnaC_stLKAEnaCSyn : Outport  Port=2
  wires:
  EnaC_bsInInfoSyn/1 -> LKA Own Condition (LKAOwnC)/2(LKAOwnC_bsInInfoSyn), Driver Intent Condition (DrvInttC)/1(DrvInttC_bsInInfoSyn), Lane Condition (LaneC)/1(LaneC_bsInInfoSyn), Vehicle State Condition (VehStateC)/2(VehStateC_bsInInfoSyn)
  Vehicle State Condition (VehStateC)/1(VehStateC_stVehStateCSyn) -> Enable Condition Synthesis (EnaCSyn)/2(EnaCSyn_stVehStateC)
  Lane Condition (LaneC)/1(LaneC_stLanCSyn) -> Enable Condition Synthesis (EnaCSyn)/3(EnaCSyn_stLaneC)
  Driver Intent Condition (DrvInttC)/1(DrvInttC_stDrvInttCSyn) -> Enable Condition Synthesis (EnaCSyn)/4(EnaCSyn_stDrvInttC)
  LDW Own Condition (LDWOwnC)/1(LDWOwnC_stLDWOwnCSyn) -> Enable Condition Synthesis (EnaCSyn)/5(EnaCSyn_stLDWOwnC)
  LKA Own Condition (LKAOwnC)/1(LKAOwnC_tfLKAOwnCSyn) -> Enable Condition Synthesis (EnaCSyn)/6(EnaCSyn_stLKAOwnC)
  Enable Condition Synthesis (EnaCSyn)/1(EnaCSyn_stLDWEnaCSyn) -> EnaC_stLDWEnaCSyn/1
  EnaC_bsLLClb/1 -> LKA Own Condition (LKAOwnC)/3(LKAOwnC_bsLLClb), LDW Own Condition (LDWOwnC)/4(LDWOwnC_bsLLClb), Driver Intent Condition (DrvInttC)/2(DrvInttC_bsLLSMConClb), Lane Condition (LaneC)/4(LaneC_bsLLSMConClb), Vehicle State Condition (VehStateC)/3(VehStateC_bsLLClb)
  EnaC_stDACMode/1 -> Vehicle State Condition (VehStateC)/1(VehStateC_stDACMode), LKA Own Condition (LKAOwnC)/1(LKAOwnC_stDACMode), LDW Own Condition (LDWOwnC)/1(LDWOwnC_stDACMode), Enable Condition Synthesis (EnaCSyn)/1(EnaCSyn_stDACMode)
  Enable Condition Synthesis (EnaCSyn)/2(EnaCSyn_stLKAEnaCSyn) -> EnaC_stLKAEnaCSyn/1  "ENABLE"
  EnaC_bsLKAInPInfo/1 -> Bus Selector/1
  Bus Selector/1 -> LDW Own Condition (LDWOwnC)/2(LDWOwnC_LaneWidth), LKA Own Condition (LKAOwnC)/5(LKAOwnC_LaneWidth), Lane Condition (LaneC)/2(LaneC_LaneWidth)  "<LaneWidth>"
  Bus Selector/2 -> Lane Condition (LaneC)/3(LaneC_crPrvwCrvt)  "<crPrvwCrvt>"
  Bus Selector/3 -> LKA Own Condition (LKAOwnC)/4(LKAOwnC_bsTTLCInfo)  "<bsTTLCInfo>"
  Bus Selector/4 -> LKA Own Condition (LKAOwnC)/6(LKAOwnC_bsDvtInfo), LDW Own Condition (LDWOwnC)/3(LDWOwnC_bsDvtInfo)  "<bsDvtInfo>"

== system LKAS_AutoSave_DF_20211230_1703/LKAS/LL/LLOn/LL State Determination (LLStateDet)/LL State Machine Conditions (LLSMCon)/Fault Condition (FaultC) ==
  FaultC_bsInInfoSyn : Inport
  FaultC_bsLLClb : Inport  Port=2
  FaultC_SignalFault : Inport  Port=3
  Bus Selector2 : BusSelector  OutputSignals=bsEPSInfo.EPS_LKA_State
  Bus Selector3 : BusSelector  OutputSignals=bsLaneInfo.Fusion_AdditionalInf.Carema_Status
  Bus Selector5 : BusSelector  OutputSignals=bsConstantClb.LKA_SampleTime
  Bus Selector6 : BusSelector  OutputSignals=LKAS_BSWDTC_Status
  Compare To Constant{1,3..12} (11 alike) : simulink/Logic and Bit Operations/Compare To Constant  relop===  const=1  OutDataTypeStr=boolean
  Compare To Constant14 : simulink/Logic and Bit Operations/Compare To Constant  relop===  const=4  OutDataTypeStr=boolean
  Compare To Constant2 : simulink/Logic and Bit Operations/Compare To Constant  relop===  const=3  OutDataTypeStr=boolean
  Count_5s1 : Subsystem
  Count_5s2 : Subsystem
  Count_5s3 : Subsystem
  Demux : Demux  Outputs=11
  Logical Operator1 : Logic  Operator=OR  Inputs=9  AllPortsSameDT=off  OutDataTypeStr=boolean
  Logical Operator10 : Logic  Operator=OR  AllPortsSameDT=off  OutDataTypeStr=boolean
  Logical Operator8 : Logic  Operator=OR  Inputs=3  AllPortsSameDT=off  OutDataTypeStr=boolean
  FaultC_stLDWFaultCSyn : Outport
  FaultC_stLKAFaultCSyn : Outport  Port=2
  wires:
  Logical Operator1/1 -> Count_5s3/Enable
  Count_5s2/1(Out) -> Logical Operator10/2, Logical Operator8/2  "Camera_Fault"
  [SampleTime] -> Count_5s2/1(SampleTime)
  Compare To Constant2/1 -> Count_5s2/Enable  "Camera_Fault"
  Compare To Constant14/1 -> Count_5s1/Enable  "EPS_State_For_LKA_Fault"
  Count_5s1/1(Out) -> Logical Operator8/3  "EPS_Fault"
  Logical Operator8/1 -> FaultC_stLKAFaultCSyn/1  "LKA_Fault"
  Logical Operator10/1 -> FaultC_stLDWFaultCSyn/1  "LDW_Fault"
  FaultC_bsInInfoSyn/1 -> Bus Selector3/1, Bus Selector2/1
  Bus Selector2/1 -> Compare To Constant14/1  "<EPS_LKA_State>"
  Bus Selector3/1 -> Compare To Constant2/1  "<Carema_Status>"
  Demux/1 -> Compare To Constant1/1  "CANEve_e_BusOff_PSA1CAN"
  Demux/2 -> Compare To Constant3/1  "CANEve_e_BusOff_SensorCAN"
  Demux/3 -> Compare To Constant4/1  "CANEve_e_Mute_PSA1CAN"
  Demux/6 -> Compare To Constant7/1  "CANEve_e_Node_EMS_Validity"
  Demux/5 -> Compare To Constant6/1  "CANEve_e_Node_EPS_Validity"
  Demux/4 -> Compare To Constant5/1  "CANEve_e_Node_ESC_Validity"
  Demux/10 -> Compare To Constant11/1  "CANEve_e_Node_Camera_Validity"
  Demux/11 -> Compare To Constant12/1  "BatteryVoltage"
  Demux/9 -> Compare To Constant10/1  "CANEve_e_Node_Radar_Validity"
  Demux/8 -> Compare To Constant9/1  "CANEve_e_Node_GW_Validity"
  Demux/7 -> Compare To Constant8/1  "CANEve_e_Node_TCU_Validity"
  Compare To Constant1/1 -> Logical Operator1/1
  Compare To Constant3/1 -> Logical Operator1/2
  Compare To Constant4/1 -> Logical Operator1/3
  Compare To Constant5/1 -> Logical Operator1/4
  Compare To Constant6/1 -> Logical Operator1/5
  Compare To Constant9/1 -> Logical Operator1/7
  Compare To Constant11/1 -> Logical Operator1/8
  FaultC_bsLLClb/1 -> Bus Selector5/1
  FaultC_SignalFault/1 -> Bus Selector6/1
  Count_5s3/1(Out) -> Logical Operator10/1, Logical Operator8/1  "CAN_Bus"
  Bus Selector6/1 -> Demux/1  "<LKAS_BSWDTC_Status>"
  Bus Selector5/1 -> [SampleTime]  "<LKA_SampleTime>"
  [SampleTime] -> Count_5s1/1(SampleTime)
  [SampleTime] -> Count_5s3/1(SampleTime)
  Compare To Constant12/1 -> Logical Operator1/9
  Compare To Constant8/1 -> Logical Operator1/6

== system LKAS_AutoSave_DF_20211230_1703/LKAS/LL/LL Inputs Mapping/bsLaneInfo/LanesReconstruct /RoadSide Offset/Average Filter (AvrgFlt) ==
  In : Inport
  PtsNum : Inport  Port=2
  Abs : Abs
  Add1 : Sum  AccumDataTypeStr=single  OutDataTypeStr=single
  Add2 : Sum  Inputs=-+
  Add3 : Sum  Inputs=+-  AccumDataTypeStr=single  OutDataTypeStr=single
  Compare To Constant : simulink/Logic and Bit Operations/Compare To Constant  relop=>  const=0.5  OutDataTypeStr=boolean
  Constant : Constant  OutDataTypeStr=single
  Constant1 : Constant  OutDataTypeStr=single
  Divide : Product  Inputs=**
  Divide1 : Product  Inputs=**
  Divide2 : Product  Inputs=*/
  Memory : Memory  InitialCondition=-1.75  InheritSampleTime=on
  Memory1 : Memory  InitialCondition=-1.75  InheritSampleTime=on
  Saturation : Saturate  UpperLimit=10000  LowerLimit=1  OutDataTypeStr=single
      settings: AttributesFormatString="Min = %<LowerLimit>  Max = %<UpperLimit>"
  Switch : Switch  Criteria=u2 > Threshold
  Out : Outport
  wires:
  Add1/1 -> Switch/3
  Compare To Constant/1 -> Switch/2
  Abs/1 -> Compare To Constant/1
  Add3/1 -> Abs/1
  Memory1/1 -> Add3/2
  Constant1/1 -> Divide2/1
  Saturation/1 -> Divide2/2
  Memory/1 -> Divide1/2
  Divide2/1 -> Divide/2, Add2/1
  Switch/1 -> Out/1, Memory/1
  Divide1/1 -> Add1/2
  Add2/1 -> Divide1/1
  Constant/1 -> Add2/2
  Divide/1 -> Add1/1
  PtsNum/1 -> Saturation/1
  In/1 -> Divide/1, Add3/1, Switch/1, Memory1/1
